simulink model "Example_2_Closed"  (Simulink 8.3)
settings: Solver=ode45  StartTime=0.0  StopTime=30  RelTol=1e-3
libraries: simulink x1
settings Model: Creator=NeuControl  LastModifiedBy=Li Jinghao
settings DataIOCC: SignalLoggingSaveFormat=Dataset
settings DebuggingCC: UnderspecifiedInitializationDetection=Simplified  StateNameClashWarn=none
settings GRTTargetCC: CombineOutputUpdateFcns=on  GRTInterface=off

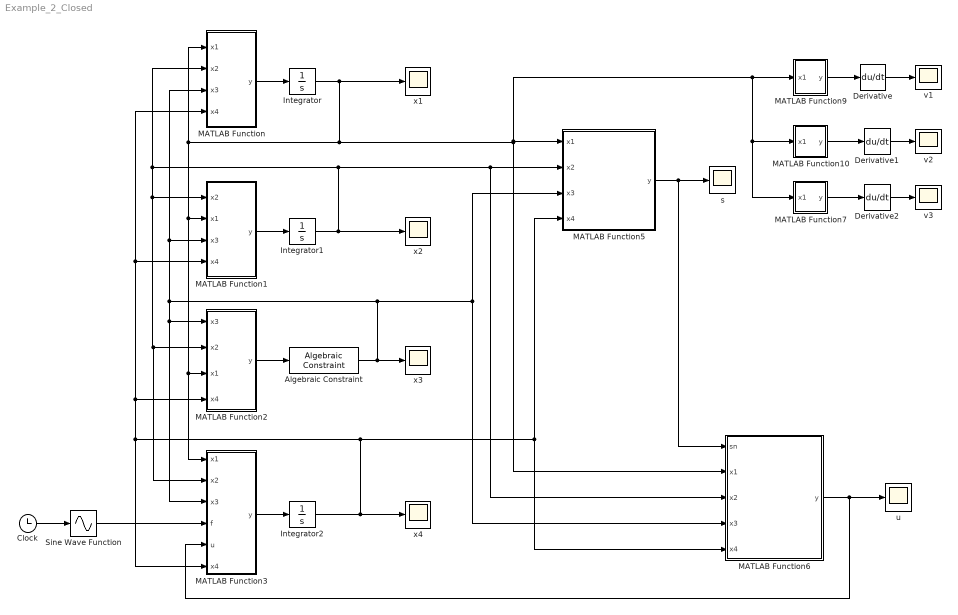
== system Example_2_Closed ==
  Algebraic Constraint : simulink/Math Operations/Algebraic Constraint  z0=0
  Clock : Clock
  Derivative : Derivative
  Derivative1 : Derivative
  Derivative2 : Derivative
  Integrator : Integrator  InitialCondition=0.5
  Integrator1 : Integrator  InitialCondition=-1
  Integrator2 : Integrator  InitialCondition=2
  MATLAB Function : MATLAB Function  TreatAsAtomicUnit=on
  MATLAB Function1 : MATLAB Function  TreatAsAtomicUnit=on
  MATLAB Function10 : MATLAB Function  TreatAsAtomicUnit=on
  MATLAB Function2 : MATLAB Function  TreatAsAtomicUnit=on
  MATLAB Function3 : MATLAB Function  TreatAsAtomicUnit=on
  MATLAB Function5 : MATLAB Function  TreatAsAtomicUnit=on
  MATLAB Function6 : MATLAB Function  TreatAsAtomicUnit=on
  MATLAB Function7 : MATLAB Function  TreatAsAtomicUnit=on
  MATLAB Function9 : MATLAB Function  TreatAsAtomicUnit=on
  Sine Wave Function : Sin  TimeSource=Use external signal  Phase=pi/2  SampleTime=0
  s : Scope
      settings: SaveName=s
  u : Scope
      settings: TimeRange=50  SaveName=u
  v1 : Scope
      settings: YMin=-0.0008  YMax=0.0007  SaveName=ScopeData3
  v2 : Scope
      settings: TimeRange=30  YMin=-0.2  YMax=0.15  SaveName=ScopeData4
  v3 : Scope
  x{1..4} (4 alike) : Scope
      x1 settings: TimeRange=30  YMin=-0.4  YMax=1  SaveName=x1
      x2 settings: SaveName=x2
      x3 settings: SaveName=x3
      x4 settings: YMin=-0.0175  YMax=0.0175  SaveName=x4
  wires:
  Integrator/1 -> MATLAB Function9/1(x1), MATLAB Function7/1(x1), MATLAB Function10/1(x1), MATLAB Function5/1(x1), MATLAB Function6/2(x1), MATLAB Function/1(x1), MATLAB Function3/1(x1), MATLAB Function2/3(x1), MATLAB Function1/2(x1), x1/1
  MATLAB Function/1(y) -> Integrator/1
  Integrator1/1 -> x2/1, MATLAB Function6/3(x2), MATLAB Function5/2(x2), MATLAB Function/2(x2), MATLAB Function3/2(x2), MATLAB Function2/2(x2), MATLAB Function1/1(x2)
  MATLAB Function1/1(y) -> Integrator1/1
  Algebraic Constraint/1 -> x3/1, MATLAB Function3/3(x3), MATLAB Function2/1(x3), MATLAB Function/3(x3), MATLAB Function1/3(x3), MATLAB Function6/4(x3), MATLAB Function5/3(x3)
  MATLAB Function2/1(y) -> Algebraic Constraint/1
  Integrator2/1 -> MATLAB Function3/6(x4), MATLAB Function/4(x4), MATLAB Function1/4(x4), MATLAB Function2/4(x4), MATLAB Function6/5(x4), MATLAB Function5/4(x4), x4/1
  MATLAB Function3/1(y) -> Integrator2/1
  Clock/1 -> Sine Wave Function/1
  Sine Wave Function/1 -> MATLAB Function3/4(f)
  MATLAB Function5/1(y) -> s/1, MATLAB Function6/1(sn)
  MATLAB Function6/1(y) -> u/1, MATLAB Function3/5(u)
  MATLAB Function9/1(y) -> Derivative/1
  Derivative/1 -> v1/1
  MATLAB Function10/1(y) -> Derivative1/1
  Derivative1/1 -> v2/1
  MATLAB Function7/1(y) -> Derivative2/1
  Derivative2/1 -> v3/1

== matlab function MATLAB Function1 ==
  data: x2 input double; x1 input double; y output double; x3 input double; x4 input double
function y = fcn(x2,x1,x3,x4)
%#codegen

gamma=1;
h1=exp(-0.5*(0.5*(x1+5))^2);
h2=exp(-0.5*(0.5*x1)^2);
h3=exp(-0.5*(0.5*(x1-5))^2);
v1=h1/(h1+h2+h3);
v2=h2/(h1+h2+h3);
v3=1-v1-v2;
A1=[-0.5 -0.5 -1 1];
A2=[0.5 -1 0 0.5];
A3=[gamma -1 1 0];
A=v1*A1+v2*A2+v3*A3;
x=[x1;x2;x3;x4];
y = A*x;

== matlab function MATLAB Function ==
  data: x1 input double; y output double; x2 input double; x3 input double; x4 input double
function y = fcn(x1,x2,x3,x4)
%#codegen

beta=-2;
gamma=1;
h1=exp(-0.5*(0.5*(x1+5))^2);
h2=exp(-0.5*(0.5*x1)^2);
h3=exp(-0.5*(0.5*(x1-5))^2);
v1=h1/(h1+h2+h3);
v2=h2/(h1+h2+h3);
v3=1-v1-v2;
A1=[-1 beta 1 -0.5];
A2=[gamma 0.5 0 1];
A3=[-1 beta 0 1];
A=v1*A1+v2*A2+v3*A3;
x=[x1;x2;x3;x4];
y = A*x;

== matlab function MATLAB Function2 ==
  data: x3 input double; x2 input double; x1 input double; y output double; x4 input double
function y = fcn(x3,x2,x1,x4)
%#codegen

h1=exp(-0.5*(0.5*(x1+5))^2);
h2=exp(-0.5*(0.5*x1)^2);
h3=exp(-0.5*(0.5*(x1-5))^2);
v1=h1/(h1+h2+h3);
v2=h2/(h1+h2+h3);
v3=1-v1-v2;
A1=[0 0 -1 1];
A2=[1 0 -1 0.5];
A3=[0 1 -1 1];
A=v1*A1+v2*A2+v3*A3;
x=[x1;x2;x3;x4];
y = A*x;

== matlab function MATLAB Function3 ==
  data: x1 input double; x2 input double; x3 input double; f input double; u input double; x4 input double; y output double
function y = fcn(x1,x2,x3,f,u,x4)
%#codegen

A=[0.5 1 -1.5 1];
x=[x1;x2;x3;x4];
y = A*x+0.5*(u+f);

== matlab function MATLAB Function5 ==
  data: x1 input double; y output double; x2 input double; x3 input double; x4 input double
function y = fcn(x1,x2,x3,x4)
%#codegen

w1=exp(-0.5*(0.5*(x1+5))^2);
w2=exp(-0.5*(0.5*x1)^2);
w3=exp(-0.5*(0.5*(x1-5))^2);
v1=w1/(w1+w2+w3);
v2=w2/(w1+w2+w3);
v3=1-v1-v2;
E=[1 0 0;...
   0 1 0;...
   0 0 0];
K1=[2.7285 -0.4465 0];
K2=[4.7377 0.3795 0];
K3=[-1.2033 1.9457 0];
K=v1*K1+v2*K2+v3*K3;
P1=[0.7104  0.2287 0;...
    0.2287  0.6717 0;...
    -2.0689 0.8671 0.4193];
P2=[1.3974  0.5890 0;...
    0.5890  0.8607 0;...
    -2.1508 0.9474 0.4594];
P3=[1.7895 0.7392  0;...
    0.7392 0.9132  0;...
    1.6678 -0.4270 0.2632];
P=v1*P1+v2*P2+v3*P3;
x123=[x1;x2;x3];
y = K*inv(P)'*E*x123+x4;

== matlab function MATLAB Function6 ==
  data: sn input double; x1 input double; y output double; x2 input double; x3 input double; x4 input double
function y = fcn(sn,x1,x2,x3,x4)
%#codegen

beta=-2;
gamma=1;
w1=exp(-0.5*(0.5*(x1+5))^2);
w2=exp(-0.5*(0.5*x1)^2);
w3=exp(-0.5*(0.5*(x1-5))^2);
v1=w1/(w1+w2+w3);
v2=w2/(w1+w2+w3);
v3=1-v1-v2;
E=[1 0 0;...
   0 1 0;...
   0 0 0];
K1=[2.7285 -0.4465 0];
K2=[4.7377 0.3795 0];
K3=[-1.2033 1.9457 0];
K=v1*K1+v2*K2+v3*K3;
P1=[0.7104  0.2287 0;...
    0.2287  0.6717 0;...
    -2.0689 0.8671 0.4193];
P2=[1.3974  0.5890 0;...
    0.5890  0.8607 0;...
    -2.1508 0.9474 0.4594];
P3=[1.7895 0.7392  0;...
    0.7392 0.9132  0;...
    1.6678 -0.4270 0.2632];
P=v1*P1+v2*P2+v3*P3;
A11=[-1   beta  1;...
     -0.5 -0.5 -1;...
     0     0   -1];
A21=[gamma 0.5  0;...
       0.5  -1  0;...
       1    0  -1];
A31=[-1   beta  0;...
    gamma  -1   1;...
     0      1  -1];
A1=v1*A11+v2*A21+v3*A31;
A12=[-0.5;1;1];
A22=[1;0.5;0.5];
A32=[1;0;1];
A2=v1*A12+v2*A22+v3*A32;
A3=[0.5 1 -1.5];
A4=1;
x123=[x1;x2;x3];
B1=0.5;
bf=1;
bx1=1;
psi1=0.1;
psi2=0.15;
psi3=0.2;
rho1=0.0001;
kappa=0.5;

rho=norm(B1)*bf+(psi1*norm(K1*inv(P)'*E)+psi2*norm(K2*inv(P)'*E)...
    +psi3*norm(K3*inv(P)'*E)+psi1*norm(K*inv(P)'*P1'*inv(P)'*E)...
    +psi2*norm(K*inv(P)'*P2'*inv(P)'*E)...
    +psi3*norm(K*inv(P)'*P3'*inv(P)'*E))*bx1+rho1;

y = -inv(B1)*((K*inv(P)'*A1+A3+kappa*K*inv(P)'*E)*x123+...
    (K*inv(P)'*A2+A4+kappa)*x4+rho*sn/(norm(sn)));

== matlab function MATLAB Function7 ==
  data: x1 input double; y output double
function y = fcn(x1)
%#codegen

h1=exp(-0.5*(0.5*(x1+5))^2);
h2=exp(-0.5*(0.5*x1)^2);
h3=exp(-0.5*(0.5*(x1-5))^2);
v1=h1/(h1+h2+h3);
v2=h2/(h1+h2+h3);
v3=1-v1-v2;

y = v3;

== matlab function MATLAB Function9 ==
  data: x1 input double; y output double
function y = fcn(x1)
%#codegen

h1=exp(-0.5*(0.5*(x1+5))^2);
h2=exp(-0.5*(0.5*x1)^2);
h3=exp(-0.5*(0.5*(x1-5))^2);
v1=h1/(h1+h2+h3);
v2=h2/(h1+h2+h3);
v3=1-v1-v2;

y = v1;

== matlab function MATLAB Function10 ==
  data: x1 input double; y output double
function y = fcn(x1)
%#codegen

h1=exp(-0.5*(0.5*(x1+5))^2);
h2=exp(-0.5*(0.5*x1)^2);
h3=exp(-0.5*(0.5*(x1-5))^2);
v1=h1/(h1+h2+h3);
v2=h2/(h1+h2+h3);
v3=1-v1-v2;

y = v2;
